simulink model "Adp_Lgt_SytmV2"  (R2021a)
settings: Solver=FixedStepDiscrete  StartTime=0.0  StopTime=1149  FixedStep=1  RelTol=1e-3
libraries: simulink x7
(part 1 of 2)
settings Model: Creator=Akshy  LastModifiedBy=abc
settings OptimizationCC: DefaultParameterBehavior=Inlined  UseDivisionForNetSlopeComputation=on  EnhancedBackFolding=on  PassReuseOutputArgsAs=Individual arguments  ZeroExternalMemoryAtStartup=off  ZeroInternalMemoryAtStartup=off  InitFltsAndDblsToZero=on  OptimizeBlockOrder=speed  DifferentSizesBufferReuse=on  OptimizationCustomize=off  EfficientTunableParamExpr=on
settings DebuggingCC: SignalInfNanChecking=warning  CheckMatrixSingularityMsg=error  IntegerOverflowMsg=error  ParameterTunabilityLossMsg=error  UniqueDataStoreMsg=warning  AssertControl=DisableAll  StrictBusMsg=ErrorOnBusTreatedAsVector  SFUndirectedBroadcastEventsDiag=error  IntegerSaturationMsg=error
settings SFSimCC: CompileTimeRecursionLimit=0  EnableRuntimeRecursion=off  MATLABDynamicMemAlloc=off
settings RTWCC: SystemTargetFile=ert.tlc  GenCodeOnly=on  TemplateMakefile=ert_default_tmf  GenerateReport=on  Toolchain=MinGW64 | gmake (64-bit Windows)  IncludeHyperlinkInReport=on  GenerateTraceInfo=on  GenerateTraceReportSl=on  GenerateTraceReportSf=on
settings CodeAppCC: ForceParamTrailComments=on  IgnoreCustomStorageClasses=off  OperatorAnnotations=on  SimulinkDataObjDesc=on  SFDataObjDesc=on  MATLABFcnDesc=on  InsertBlockDesc=on
settings ERTTargetCC: TargetLangStandard=C99 (ISO)  UtilityFuncGeneration=Shared location  GenerateSampleERTMain=on  SupportAbsoluteTime=off  ParenthesesLevel=Maximum  CastingMode=Standards  GenerateSharedConstants=off  InlinedParameterPlacement=NonHierarchical  ERTCustomFileTemplate=example_file_process.tlc  EnableSignedLeftShifts=off  EnableSignedRightShifts=off
settings ConfigComp: CovMetricSettings=dcmwe  PSVerificationSettings=PrjConfigAndMisraC2012  PSAutoStubLUT=on

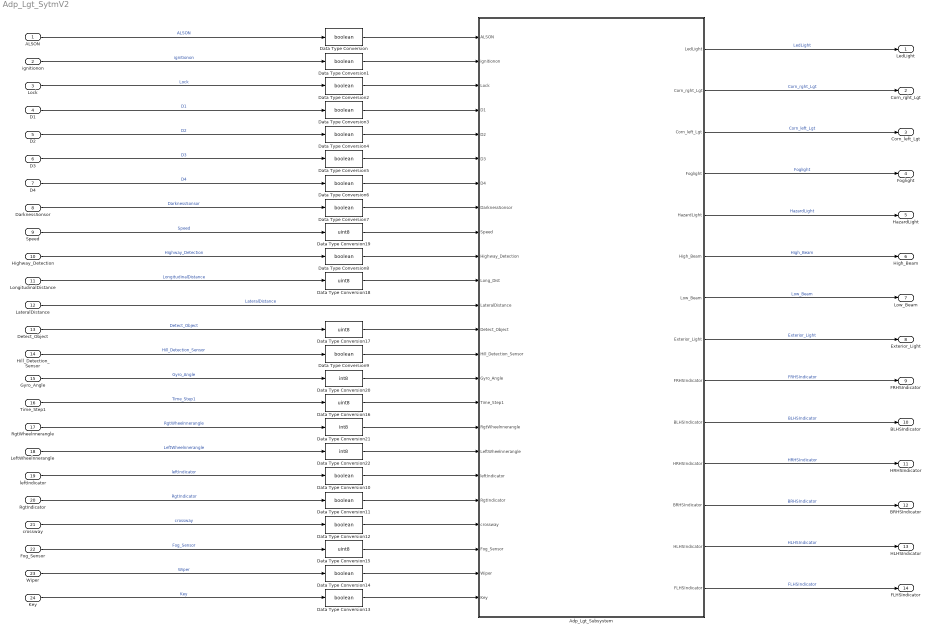
== system Adp_Lgt_SytmV2 ==
  ALSON : Inport
  ignitionon : Inport  Port=2
  Lock : Inport  Port=3
  D1 : Inport  Port=4
  D2 : Inport  Port=5
  D3 : Inport  Port=6
  D4 : Inport  Port=7
  DarknessSonsor : Inport  Port=8
  Speed : Inport  Port=9
  Highway_Detection : Inport  Port=10
  LongitudinalDistance : Inport  Port=11
  LateralDistance : Inport  Port=12
  Detect_Object : Inport  Port=13
  Hill_Detection_Sensor : Inport  Port=14
  Gyro_Angle : Inport  Port=15
  Time_Step1 : Inport  Port=16
  RgtWheelnnerangle : Inport  Port=17
  LeftWheelnnerangle : Inport  Port=18
  leftIndicator : Inport  Port=19
  RgtIndicator : Inport  Port=20
  crossway : Inport  Port=21
  Fog_Sensor : Inport  Port=22
  Wiper : Inport  Port=23
  Key : Inport  Port=24
  Adp_Lgt_Subsystem : Subsystem  TreatAsAtomicUnit=on
  Data Type Conversion{,1..14} (15 alike) : DataTypeConversion  OutDataTypeStr=boolean
  Data Type Conversion{15..19} (5 alike) : DataTypeConversion  OutDataTypeStr=uint8
  Data Type Conversion20 : DataTypeConversion  OutDataTypeStr=int8
  Data Type Conversion21 : DataTypeConversion  OutDataTypeStr=int8
  Data Type Conversion22 : DataTypeConversion  OutDataTypeStr=int8
  LedLight : Outport
  Corn_rght_Lgt : Outport  Port=2
  Corn_left_Lgt : Outport  Port=3
  Foglight : Outport  Port=4
  HazardLight : Outport  Port=5
  High_Beam : Outport  Port=6
  Low_Beam : Outport  Port=7
  Exterior_Light : Outport  Port=8
  FRHSIndicator : Outport  Port=9
  BLHSIndicator : Outport  Port=10
  HRHSIndicator : Outport  Port=11
  BRHSIndicator : Outport  Port=12
  HLHSIndicator : Outport  Port=13
  FLHSIndicator : Outport  Port=14
  wires:
  Adp_Lgt_Subsystem/13(HLHSIndicator) -> HLHSIndicator/1  "HLHSIndicator"
  Adp_Lgt_Subsystem/11(HRHSIndicator) -> HRHSIndicator/1  "HRHSIndicator"
  Adp_Lgt_Subsystem/9(FRHSIndicator) -> FRHSIndicator/1  "FRHSIndicator"
  Adp_Lgt_Subsystem/12(BRHSIndicator) -> BRHSIndicator/1  "BRHSIndicator"
  Adp_Lgt_Subsystem/4(Foglight) -> Foglight/1  "Foglight"
  Adp_Lgt_Subsystem/8(Exterior_Light) -> Exterior_Light/1  "Exterior_Light"
  Adp_Lgt_Subsystem/3(Corn_left_Lgt) -> Corn_left_Lgt/1  "Corn_left_Lgt"
  Adp_Lgt_Subsystem/6(High_Beam) -> High_Beam/1  "High_Beam"
  Adp_Lgt_Subsystem/10(BLHSIndicator) -> BLHSIndicator/1  "BLHSIndicator"
  Adp_Lgt_Subsystem/7(Low_Beam) -> Low_Beam/1  "Low_Beam"
  Adp_Lgt_Subsystem/14(FLHSIndicator) -> FLHSIndicator/1  "FLHSIndicator"
  Adp_Lgt_Subsystem/2(Corn_rght_Lgt) -> Corn_rght_Lgt/1  "Corn_rght_Lgt"
  Adp_Lgt_Subsystem/1(LedLight) -> LedLight/1  "LedLight"
  Adp_Lgt_Subsystem/5(HazardLight) -> HazardLight/1  "HazardLight"
  Data Type Conversion/1 -> Adp_Lgt_Subsystem/1(ALSON)
  Data Type Conversion1/1 -> Adp_Lgt_Subsystem/2(ignitionon)
  Data Type Conversion2/1 -> Adp_Lgt_Subsystem/3(Lock)
  Data Type Conversion3/1 -> Adp_Lgt_Subsystem/4(D1)
  Data Type Conversion4/1 -> Adp_Lgt_Subsystem/5(D2)
  Data Type Conversion5/1 -> Adp_Lgt_Subsystem/6(D3)
  Data Type Conversion6/1 -> Adp_Lgt_Subsystem/7(D4)
  Data Type Conversion7/1 -> Adp_Lgt_Subsystem/8(DarknessSonsor)
  Data Type Conversion8/1 -> Adp_Lgt_Subsystem/10(Highway_Detection)
  Data Type Conversion9/1 -> Adp_Lgt_Subsystem/14(Hill_Detection_Sensor)
  Data Type Conversion10/1 -> Adp_Lgt_Subsystem/19(leftIndicator)
  Data Type Conversion11/1 -> Adp_Lgt_Subsystem/20(RgtIndicator)
  Data Type Conversion12/1 -> Adp_Lgt_Subsystem/21(crossway)
  Data Type Conversion13/1 -> Adp_Lgt_Subsystem/24(Key)
  Data Type Conversion14/1 -> Adp_Lgt_Subsystem/23(Wiper)
  Data Type Conversion15/1 -> Adp_Lgt_Subsystem/22(Fog_Sensor)
  Data Type Conversion16/1 -> Adp_Lgt_Subsystem/16(Time_Step1)
  Data Type Conversion17/1 -> Adp_Lgt_Subsystem/13(Detect_Object)
  Data Type Conversion18/1 -> Adp_Lgt_Subsystem/11(Long_Dist)
  Data Type Conversion19/1 -> Adp_Lgt_Subsystem/9(Speed)
  Data Type Conversion20/1 -> Adp_Lgt_Subsystem/15(Gyro_Angle)
  Data Type Conversion21/1 -> Adp_Lgt_Subsystem/17(RgtWheelnnerangle)
  Data Type Conversion22/1 -> Adp_Lgt_Subsystem/18(LeftWheelnnerangle)
  Detect_Object/1 -> Data Type Conversion17/1  "Detect_Object"
  Time_Step1/1 -> Data Type Conversion16/1  "Time_Step1"
  leftIndicator/1 -> Data Type Conversion10/1  "leftIndicator"
  Wiper/1 -> Data Type Conversion14/1  "Wiper"
  Hill_Detection_Sensor/1 -> Data Type Conversion9/1  "Hill_Detection_Sensor"
  Fog_Sensor/1 -> Data Type Conversion15/1  "Fog_Sensor"
  Gyro_Angle/1 -> Data Type Conversion20/1  "Gyro_Angle"
  crossway/1 -> Data Type Conversion12/1  "crossway"
  LeftWheelnnerangle/1 -> Data Type Conversion22/1  "LeftWheelnnerangle"
  RgtWheelnnerangle/1 -> Data Type Conversion21/1  "RgtWheelnnerangle"
  Highway_Detection/1 -> Data Type Conversion8/1  "Highway_Detection"
  D3/1 -> Data Type Conversion5/1  "D3"
  RgtIndicator/1 -> Data Type Conversion11/1  "RgtIndicator"
  LateralDistance/1 -> Adp_Lgt_Subsystem/12(LateralDistance)  "LateralDistance"
  LongitudinalDistance/1 -> Data Type Conversion18/1  "LongitudinalDistance"
  Lock/1 -> Data Type Conversion2/1  "Lock"
  DarknessSonsor/1 -> Data Type Conversion7/1  "DarknessSonsor"
  ALSON/1 -> Data Type Conversion/1  "ALSON"
  D2/1 -> Data Type Conversion4/1  "D2"
  ignitionon/1 -> Data Type Conversion1/1  "ignitionon"
  D4/1 -> Data Type Conversion6/1  "D4"
  Key/1 -> Data Type Conversion13/1  "Key"
  D1/1 -> Data Type Conversion3/1  "D1"
  Speed/1 -> Data Type Conversion19/1  "Speed"

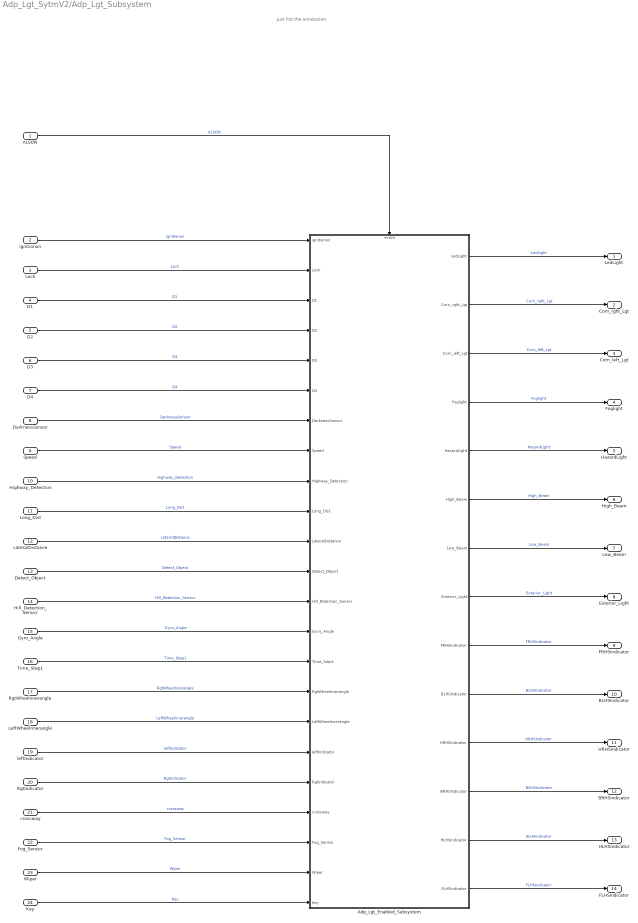
== system Adp_Lgt_SytmV2/Adp_Lgt_Subsystem ==
  note: Just Put the annotation
  ALSON : Inport  OutDataTypeStr=boolean
  ignitionon : Inport  Port=2  OutDataTypeStr=boolean
  Lock : Inport  Port=3  OutDataTypeStr=boolean
  D1 : Inport  Port=4  OutDataTypeStr=boolean
  D2 : Inport  Port=5  OutDataTypeStr=boolean
  D3 : Inport  Port=6  OutDataTypeStr=boolean
  D4 : Inport  Port=7  OutDataTypeStr=boolean
  DarknessSonsor : Inport  Port=8  OutDataTypeStr=boolean
  Speed : Inport  Port=9  OutDataTypeStr=uint8
  Highway_Detection : Inport  Port=10  OutDataTypeStr=boolean
  Long_Dist : Inport  Port=11  OutDataTypeStr=uint8
  LateralDistance : Inport  Port=12  OutDataTypeStr=double
  Detect_Object : Inport  Port=13  OutDataTypeStr=uint8
  Hill_Detection_Sensor : Inport  Port=14  OutDataTypeStr=boolean
  Gyro_Angle : Inport  Port=15  OutDataTypeStr=int8
  Time_Step1 : Inport  Port=16  OutDataTypeStr=uint8
  RgtWheelnnerangle : Inport  Port=17  OutDataTypeStr=int8
  LeftWheelnnerangle : Inport  Port=18  OutDataTypeStr=int8
  leftIndicator : Inport  Port=19  OutDataTypeStr=boolean
  RgtIndicator : Inport  Port=20  OutDataTypeStr=boolean
  crossway : Inport  Port=21  OutDataTypeStr=boolean
  Fog_Sensor : Inport  Port=22  OutDataTypeStr=uint8
  Wiper : Inport  Port=23
  Key : Inport  Port=24  OutDataTypeStr=boolean
  Adp_Lgt_Enabled_Subsystem : Subsystem  TreatAsAtomicUnit=on
  LedLight : Outport
  Corn_rght_Lgt : Outport  Port=2
  Corn_left_Lgt : Outport  Port=3
  Foglight : Outport  Port=4
  HazardLight : Outport  Port=5
  High_Beam : Outport  Port=6
  Low_Beam : Outport  Port=7
  Exterior_Light : Outport  Port=8
  FRHSIndicator : Outport  Port=9
  BLHSIndicator : Outport  Port=10
  HRHSIndicator : Outport  Port=11
  BRHSIndicator : Outport  Port=12
  HLHSIndicator : Outport  Port=13
  FLHSIndicator : Outport  Port=14
  wires:
  LeftWheelnnerangle/1 -> Adp_Lgt_Enabled_Subsystem/17(LeftWheelnnerangle)  "LeftWheelnnerangle"
  Detect_Object/1 -> Adp_Lgt_Enabled_Subsystem/12(Detect_Object)  "Detect_Object"
  D4/1 -> Adp_Lgt_Enabled_Subsystem/6(D4)  "D4"
  RgtWheelnnerangle/1 -> Adp_Lgt_Enabled_Subsystem/16(RgtWheelnnerangle)  "RgtWheelnnerangle"
  LateralDistance/1 -> Adp_Lgt_Enabled_Subsystem/11(LateralDistance)  "LateralDistance"
  Adp_Lgt_Enabled_Subsystem/1(LedLight) -> LedLight/1  "LedLight"
  Adp_Lgt_Enabled_Subsystem/2(Corn_rght_Lgt) -> Corn_rght_Lgt/1  "Corn_rght_Lgt"
  Adp_Lgt_Enabled_Subsystem/4(Foglight) -> Foglight/1  "Foglight"
  crossway/1 -> Adp_Lgt_Enabled_Subsystem/20(crossway)  "crossway"
  RgtIndicator/1 -> Adp_Lgt_Enabled_Subsystem/19(RgtIndicator)  "RgtIndicator"
  Highway_Detection/1 -> Adp_Lgt_Enabled_Subsystem/9(Highway_Detection)  "Highway_Detection"
  leftIndicator/1 -> Adp_Lgt_Enabled_Subsystem/18(leftIndicator)  "leftIndicator"
  DarknessSonsor/1 -> Adp_Lgt_Enabled_Subsystem/7(DarknessSonsor)  "DarknessSonsor"
  ignitionon/1 -> Adp_Lgt_Enabled_Subsystem/1(ignitionon)  "ignitionon"
  Speed/1 -> Adp_Lgt_Enabled_Subsystem/8(Speed)  "Speed"
  Adp_Lgt_Enabled_Subsystem/5(HazardLight) -> HazardLight/1  "HazardLight"
  Time_Step1/1 -> Adp_Lgt_Enabled_Subsystem/15(Time_Step1)  "Time_Step1"
  Fog_Sensor/1 -> Adp_Lgt_Enabled_Subsystem/21(Fog_Sensor)  "Fog_Sensor"
  Lock/1 -> Adp_Lgt_Enabled_Subsystem/2(Lock)  "Lock"
  Long_Dist/1 -> Adp_Lgt_Enabled_Subsystem/10(Long_Dist)  "Long_Dist"
  D1/1 -> Adp_Lgt_Enabled_Subsystem/3(D1)  "D1"
  Gyro_Angle/1 -> Adp_Lgt_Enabled_Subsystem/14(Gyro_Angle)  "Gyro_Angle"
  D3/1 -> Adp_Lgt_Enabled_Subsystem/5(D3)  "D3"
  Wiper/1 -> Adp_Lgt_Enabled_Subsystem/22(Wiper)  "Wiper"
  Adp_Lgt_Enabled_Subsystem/3(Corn_left_Lgt) -> Corn_left_Lgt/1  "Corn_left_Lgt"
  D2/1 -> Adp_Lgt_Enabled_Subsystem/4(D2)  "D2"
  ALSON/1 -> Adp_Lgt_Enabled_Subsystem/Enable  "ALSON"
  Key/1 -> Adp_Lgt_Enabled_Subsystem/23(Key)  "Key"
  Adp_Lgt_Enabled_Subsystem/9(FRHSIndicator) -> FRHSIndicator/1  "FRHSIndicator"
  Adp_Lgt_Enabled_Subsystem/10(BLHSIndicator) -> BLHSIndicator/1  "BLHSIndicator"
  Adp_Lgt_Enabled_Subsystem/11(HRHSIndicator) -> HRHSIndicator/1  "HRHSIndicator"
  Adp_Lgt_Enabled_Subsystem/14(FLHSIndicator) -> FLHSIndicator/1  "FLHSIndicator"
  Adp_Lgt_Enabled_Subsystem/8(Exterior_Light) -> Exterior_Light/1  "Exterior_Light"
  Adp_Lgt_Enabled_Subsystem/12(BRHSIndicator) -> BRHSIndicator/1  "BRHSIndicator"
  Adp_Lgt_Enabled_Subsystem/13(HLHSIndicator) -> HLHSIndicator/1  "HLHSIndicator"
  Adp_Lgt_Enabled_Subsystem/6(High_Beam) -> High_Beam/1  "High_Beam"
  Adp_Lgt_Enabled_Subsystem/7(Low_Beam) -> Low_Beam/1  "Low_Beam"
  Hill_Detection_Sensor/1 -> Adp_Lgt_Enabled_Subsystem/13(Hill_Detection_Sensor)  "Hill_Detection_Sensor"

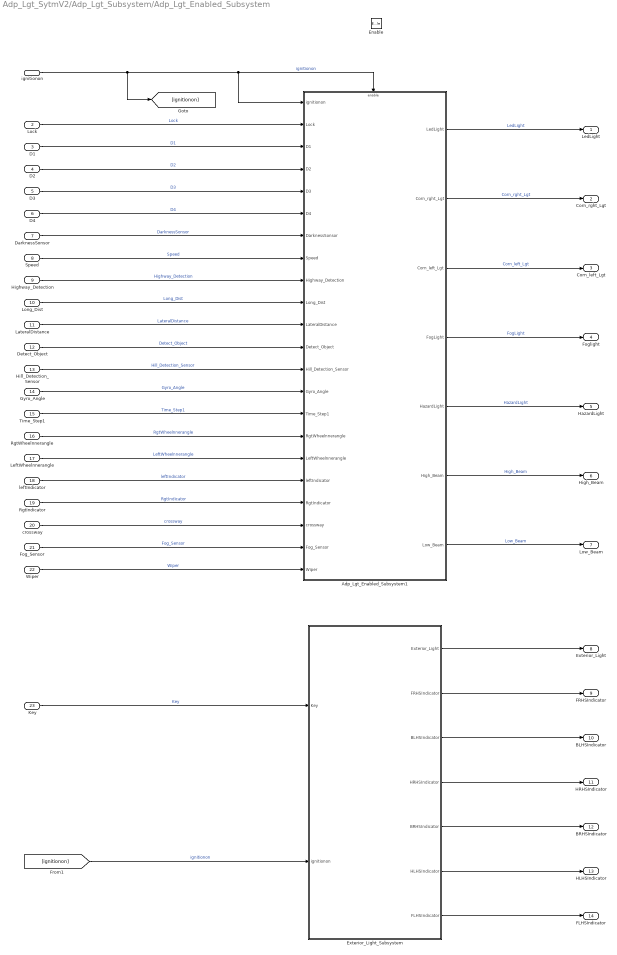
== system Adp_Lgt_SytmV2/Adp_Lgt_Subsystem/Adp_Lgt_Enabled_Subsystem ==
  ignitionon : Inport
  Lock : Inport  Port=2
  D1 : Inport  Port=3
  D2 : Inport  Port=4
  D3 : Inport  Port=5  OutDataTypeStr=boolean
  D4 : Inport  Port=6
  DarknessSonsor : Inport  Port=7
  Speed : Inport  Port=8
  Highway_Detection : Inport  Port=9
  Long_Dist : Inport  Port=10
  LateralDistance : Inport  Port=11
  Detect_Object : Inport  Port=12
  Hill_Detection_Sensor : Inport  Port=13
  Gyro_Angle : Inport  Port=14
  Time_Step1 : Inport  Port=15
  RgtWheelnnerangle : Inport  Port=16
  LeftWheelnnerangle : Inport  Port=17
  leftIndicator : Inport  Port=18
  RgtIndicator : Inport  Port=19
  crossway : Inport  Port=20
  Fog_Sensor : Inport  Port=21  OutDataTypeStr=uint8
  Wiper : Inport  Port=22
  Key : Inport  Port=23
  Enable : EnablePort
  Adp_Lgt_Enabled_Subsystem1 : Subsystem  TreatAsAtomicUnit=on
  Exterior_Light_Subsystem : Subsystem  TreatAsAtomicUnit=on
  LedLight : Outport
  Corn_rght_Lgt : Outport  Port=2
  Corn_left_Lgt : Outport  Port=3
  Foglight : Outport  Port=4
  HazardLight : Outport  Port=5
  High_Beam : Outport  Port=6
  Low_Beam : Outport  Port=7
  Exterior_Light : Outport  Port=8
  FRHSIndicator : Outport  Port=9
  BLHSIndicator : Outport  Port=10
  HRHSIndicator : Outport  Port=11
  BRHSIndicator : Outport  Port=12
  HLHSIndicator : Outport  Port=13
  FLHSIndicator : Outport  Port=14
  wires:
  D4/1 -> Adp_Lgt_Enabled_Subsystem1/6(D4)  "D4"
  DarknessSonsor/1 -> Adp_Lgt_Enabled_Subsystem1/7(DarknessSonsor)  "DarknessSonsor"
  Fog_Sensor/1 -> Adp_Lgt_Enabled_Subsystem1/21(Fog_Sensor)  "Fog_Sensor"
  Wiper/1 -> Adp_Lgt_Enabled_Subsystem1/22(Wiper)  "Wiper"
  D1/1 -> Adp_Lgt_Enabled_Subsystem1/3(D1)  "D1"
  Lock/1 -> Adp_Lgt_Enabled_Subsystem1/2(Lock)  "Lock"
  D2/1 -> Adp_Lgt_Enabled_Subsystem1/4(D2)  "D2"
  D3/1 -> Adp_Lgt_Enabled_Subsystem1/5(D3)  "D3"
  crossway/1 -> Adp_Lgt_Enabled_Subsystem1/20(crossway)  "crossway"
  Speed/1 -> Adp_Lgt_Enabled_Subsystem1/8(Speed)  "Speed"
  Highway_Detection/1 -> Adp_Lgt_Enabled_Subsystem1/9(Highway_Detection)  "Highway_Detection"
  Long_Dist/1 -> Adp_Lgt_Enabled_Subsystem1/10(Long_Dist)  "Long_Dist"
  LateralDistance/1 -> Adp_Lgt_Enabled_Subsystem1/11(LateralDistance)  "LateralDistance"
  Detect_Object/1 -> Adp_Lgt_Enabled_Subsystem1/12(Detect_Object)  "Detect_Object"
  RgtWheelnnerangle/1 -> Adp_Lgt_Enabled_Subsystem1/16(RgtWheelnnerangle)  "RgtWheelnnerangle"
  LeftWheelnnerangle/1 -> Adp_Lgt_Enabled_Subsystem1/17(LeftWheelnnerangle)  "LeftWheelnnerangle"
  leftIndicator/1 -> Adp_Lgt_Enabled_Subsystem1/18(leftIndicator)  "leftIndicator"
  RgtIndicator/1 -> Adp_Lgt_Enabled_Subsystem1/19(RgtIndicator)  "RgtIndicator"
  Adp_Lgt_Enabled_Subsystem1/4(FogLight) -> Foglight/1  "FogLight"
  Adp_Lgt_Enabled_Subsystem1/5(HazardLight) -> HazardLight/1  "HazardLight"
  Adp_Lgt_Enabled_Subsystem1/1(LedLight) -> LedLight/1  "LedLight"
  Adp_Lgt_Enabled_Subsystem1/2(Corn_rght_Lgt) -> Corn_rght_Lgt/1  "Corn_rght_Lgt"
  Adp_Lgt_Enabled_Subsystem1/3(Corn_left_Lgt) -> Corn_left_Lgt/1  "Corn_left_Lgt"
  Gyro_Angle/1 -> Adp_Lgt_Enabled_Subsystem1/14(Gyro_Angle)  "Gyro_Angle"
  Time_Step1/1 -> Adp_Lgt_Enabled_Subsystem1/15(Time_Step1)  "Time_Step1"
  Key/1 -> Exterior_Light_Subsystem/1(Key)  "Key"
  ignitionon/1 -> Adp_Lgt_Enabled_Subsystem1/Enable, Adp_Lgt_Enabled_Subsystem1/1(ignitionon), [ignitionon]  "ignitionon"
  [ignitionon] -> Exterior_Light_Subsystem/2(ignitionon)  "ignitionon"
  Adp_Lgt_Enabled_Subsystem1/6(High_Beam) -> High_Beam/1  "High_Beam"
  Adp_Lgt_Enabled_Subsystem1/7(Low_Beam) -> Low_Beam/1  "Low_Beam"
  Hill_Detection_Sensor/1 -> Adp_Lgt_Enabled_Subsystem1/13(Hill_Detection_Sensor)  "Hill_Detection_Sensor"
  Exterior_Light_Subsystem/1(Exterior_Light) -> Exterior_Light/1
  Exterior_Light_Subsystem/2(FRHSIndicator) -> FRHSIndicator/1
  Exterior_Light_Subsystem/3(BLHSIndicator) -> BLHSIndicator/1
  Exterior_Light_Subsystem/4(HRHSIndicator) -> HRHSIndicator/1
  Exterior_Light_Subsystem/5(BRHSIndicator) -> BRHSIndicator/1
  Exterior_Light_Subsystem/6(HLHSIndicator) -> HLHSIndicator/1
  Exterior_Light_Subsystem/7(FLHSIndicator) -> FLHSIndicator/1

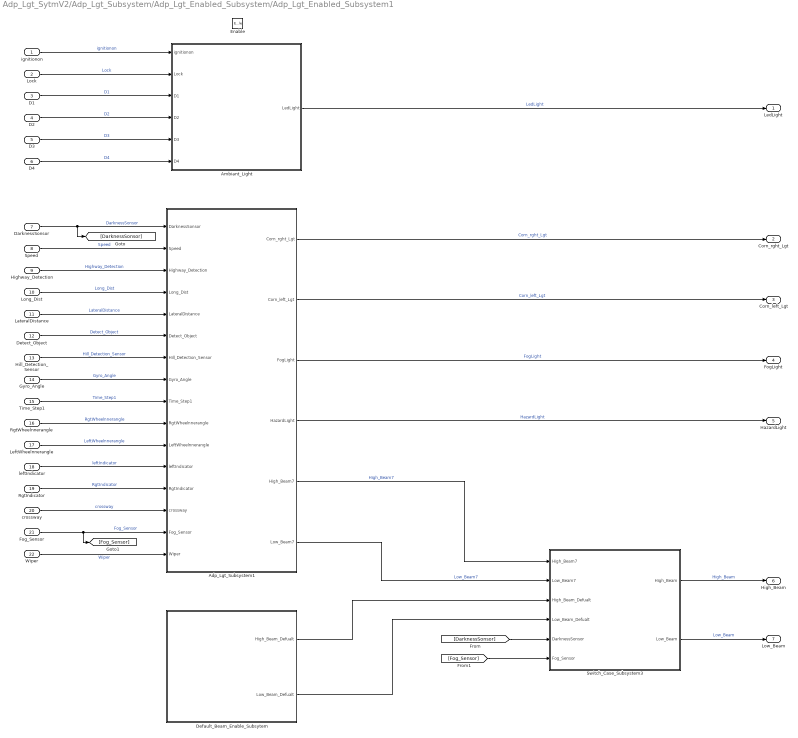
== system Adp_Lgt_SytmV2/Adp_Lgt_Subsystem/Adp_Lgt_Enabled_Subsystem/Adp_Lgt_Enabled_Subsystem1 ==
  ignitionon : Inport
  Lock : Inport  Port=2
  D1 : Inport  Port=3
  D2 : Inport  Port=4
  D3 : Inport  Port=5
  D4 : Inport  Port=6
  DarknessSonsor : Inport  Port=7
  Speed : Inport  Port=8
  Highway_Detection : Inport  Port=9
  Long_Dist : Inport  Port=10
  LateralDistance : Inport  Port=11
  Detect_Object : Inport  Port=12
  Hill_Detection_Sensor : Inport  Port=13
  Gyro_Angle : Inport  Port=14
  Time_Step1 : Inport  Port=15
  RgtWheelnnerangle : Inport  Port=16
  LeftWheelnnerangle : Inport  Port=17
  leftIndicator : Inport  Port=18
  RgtIndicator : Inport  Port=19
  crossway : Inport  Port=20
  Fog_Sensor : Inport  Port=21
  Wiper : Inport  Port=22
  Enable : EnablePort
  Adp_Lgt_Subsystem1 : Subsystem  TreatAsAtomicUnit=on
  Ambiant_Light : Subsystem  TreatAsAtomicUnit=on
  Default_Beam_Enable_Subsytem : Subsystem  TreatAsAtomicUnit=on
  Switch_Case_Subsystem3 : Subsystem  TreatAsAtomicUnit=on
  LedLight : Outport
  Corn_rght_Lgt : Outport  Port=2
  Corn_left_Lgt : Outport  Port=3
  FogLight : Outport  Port=4
  HazardLight : Outport  Port=5
  High_Beam : Outport  Port=6
  Low_Beam : Outport  Port=7
  wires:
  D1/1 -> Ambiant_Light/3(D1)  "D1"
  D3/1 -> Ambiant_Light/5(D3)  "D3"
  D4/1 -> Ambiant_Light/6(D4)  "D4"
  Ambiant_Light/1(LedLight) -> LedLight/1  "LedLight"
  Lock/1 -> Ambiant_Light/2(Lock)  "Lock"
  D2/1 -> Ambiant_Light/4(D2)  "D2"
  ignitionon/1 -> Ambiant_Light/1(ignitionon)  "ignitionon"
  Default_Beam_Enable_Subsytem/2(Low_Beam_Defualt) -> Switch_Case_Subsystem3/4(Low_Beam_Defualt)
  Default_Beam_Enable_Subsytem/1(High_Beam_Defualt) -> Switch_Case_Subsystem3/3(High_Beam_Defualt)
  DarknessSonsor/1 -> [DarknessSonsor], Adp_Lgt_Subsystem1/1(DarknessSonsor)  "DarknessSonsor"
  Speed/1 -> Adp_Lgt_Subsystem1/2(Speed)  "Speed"
  Highway_Detection/1 -> Adp_Lgt_Subsystem1/3(Highway_Detection)  "Highway_Detection"
  Long_Dist/1 -> Adp_Lgt_Subsystem1/4(Long_Dist)  "Long_Dist"
  LateralDistance/1 -> Adp_Lgt_Subsystem1/5(LateralDistance)  "LateralDistance"
  Detect_Object/1 -> Adp_Lgt_Subsystem1/6(Detect_Object)  "Detect_Object"
  Hill_Detection_Sensor/1 -> Adp_Lgt_Subsystem1/7(Hill_Detection_Sensor)  "Hill_Detection_Sensor"
  Gyro_Angle/1 -> Adp_Lgt_Subsystem1/8(Gyro_Angle)  "Gyro_Angle"
  Time_Step1/1 -> Adp_Lgt_Subsystem1/9(Time_Step1)  "Time_Step1"
  RgtWheelnnerangle/1 -> Adp_Lgt_Subsystem1/10(RgtWheelnnerangle)  "RgtWheelnnerangle"
  LeftWheelnnerangle/1 -> Adp_Lgt_Subsystem1/11(LeftWheelnnerangle)  "LeftWheelnnerangle"
  leftIndicator/1 -> Adp_Lgt_Subsystem1/12(leftIndicator)  "leftIndicator"
  RgtIndicator/1 -> Adp_Lgt_Subsystem1/13(RgtIndicator)  "RgtIndicator"
  crossway/1 -> Adp_Lgt_Subsystem1/14(crossway)  "crossway"
  Fog_Sensor/1 -> [Fog_Sensor], Adp_Lgt_Subsystem1/15(Fog_Sensor)  "Fog_Sensor"
  Wiper/1 -> Adp_Lgt_Subsystem1/16(Wiper)  "Wiper"
  Adp_Lgt_Subsystem1/5(High_Beam7) -> Switch_Case_Subsystem3/1(High_Beam7)  "High_Beam7"
  Adp_Lgt_Subsystem1/6(Low_Beam7) -> Switch_Case_Subsystem3/2(Low_Beam7)  "Low_Beam7"
  Adp_Lgt_Subsystem1/1(Corn_rght_Lgt) -> Corn_rght_Lgt/1  "Corn_rght_Lgt"
  Adp_Lgt_Subsystem1/2(Corn_left_Lgt) -> Corn_left_Lgt/1  "Corn_left_Lgt"
  Adp_Lgt_Subsystem1/3(FogLight) -> FogLight/1  "FogLight"
  Adp_Lgt_Subsystem1/4(HazardLight) -> HazardLight/1  "HazardLight"
  [DarknessSonsor] -> Switch_Case_Subsystem3/5(DarknessSonsor)
  [Fog_Sensor] -> Switch_Case_Subsystem3/6(Fog_Sensor)
  Switch_Case_Subsystem3/1(High_Beam) -> High_Beam/1  "High_Beam"
  Switch_Case_Subsystem3/2(Low_Beam) -> Low_Beam/1  "Low_Beam"

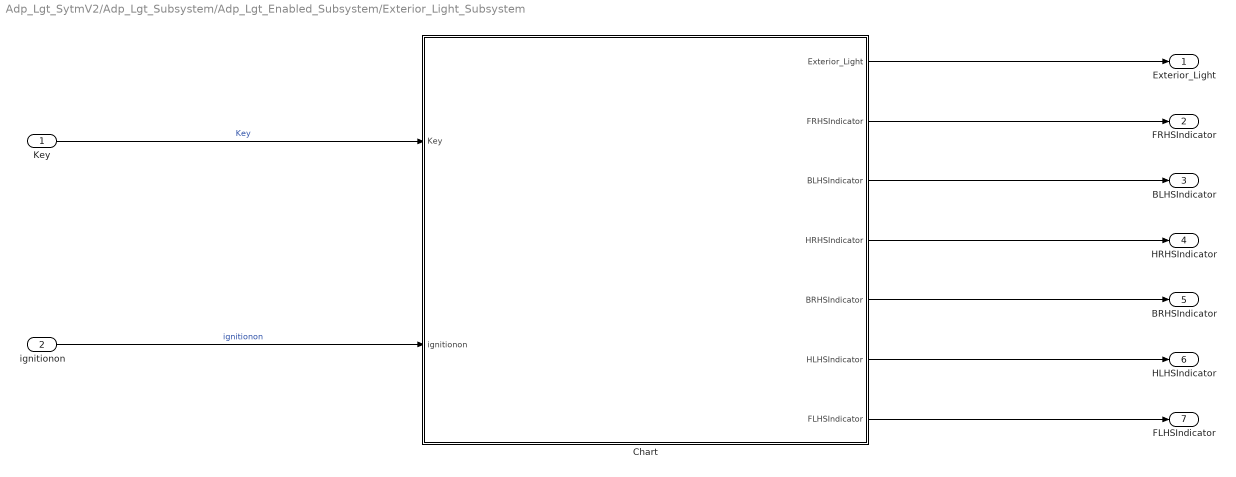
== system Adp_Lgt_SytmV2/Adp_Lgt_Subsystem/Adp_Lgt_Enabled_Subsystem/Exterior_Light_Subsystem ==
  Key : Inport
  ignitionon : Inport  Port=2
  Chart : Stateflow chart  TreatAsAtomicUnit=on
  Exterior_Light : Outport
  FRHSIndicator : Outport  Port=2
  BLHSIndicator : Outport  Port=3
  HRHSIndicator : Outport  Port=4
  BRHSIndicator : Outport  Port=5
  HLHSIndicator : Outport  Port=6
  FLHSIndicator : Outport  Port=7
  wires:
  Chart/6(HLHSIndicator) -> HLHSIndicator/1
  Key/1 -> Chart/1(Key)  "Key"
  Chart/1(Exterior_Light) -> Exterior_Light/1
  Chart/7(FLHSIndicator) -> FLHSIndicator/1
  Chart/2(FRHSIndicator) -> FRHSIndicator/1
  Chart/5(BRHSIndicator) -> BRHSIndicator/1
  Chart/3(BLHSIndicator) -> BLHSIndicator/1
  Chart/4(HRHSIndicator) -> HRHSIndicator/1
  ignitionon/1 -> Chart/2(ignitionon)  "ignitionon"

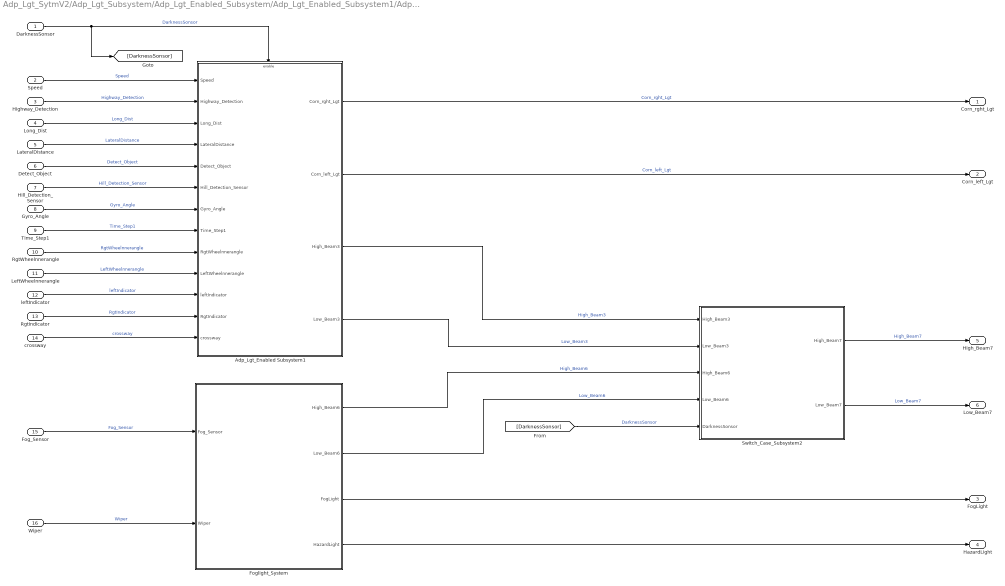
== system Adp_Lgt_SytmV2/Adp_Lgt_Subsystem/Adp_Lgt_Enabled_Subsystem/Adp_Lgt_Enabled_Subsystem1/Adp_Lgt_Subsystem1 ==
  DarknessSonsor : Inport
  Speed : Inport  Port=2
  Highway_Detection : Inport  Port=3
  Long_Dist : Inport  Port=4
  LateralDistance : Inport  Port=5
  Detect_Object : Inport  Port=6
  Hill_Detection_Sensor : Inport  Port=7
  Gyro_Angle : Inport  Port=8
  Time_Step1 : Inport  Port=9
  RgtWheelnnerangle : Inport  Port=10
  LeftWheelnnerangle : Inport  Port=11
  leftIndicator : Inport  Port=12
  RgtIndicator : Inport  Port=13
  crossway : Inport  Port=14
  Fog_Sensor : Inport  Port=15
  Wiper : Inport  Port=16
  Adp_Lgt_Enabled Subsystem1 : Subsystem  TreatAsAtomicUnit=on
  Foglight_System : Subsystem  TreatAsAtomicUnit=on
  Switch_Case_Subsystem2 : Subsystem  TreatAsAtomicUnit=on
  Corn_rght_Lgt : Outport
  Corn_left_Lgt : Outport  Port=2
  FogLight : Outport  Port=3
  HazardLight : Outport  Port=4
  High_Beam7 : Outport  Port=5
  Low_Beam7 : Outport  Port=6
  wires:
  DarknessSonsor/1 -> [DarknessSonsor], Adp_Lgt_Enabled Subsystem1/Enable  "DarknessSonsor"
  RgtIndicator/1 -> Adp_Lgt_Enabled Subsystem1/12(RgtIndicator)  "RgtIndicator"
  Hill_Detection_Sensor/1 -> Adp_Lgt_Enabled Subsystem1/6(Hill_Detection_Sensor)  "Hill_Detection_Sensor"
  Wiper/1 -> Foglight_System/2(Wiper)  "Wiper"
  LateralDistance/1 -> Adp_Lgt_Enabled Subsystem1/4(LateralDistance)  "LateralDistance"
  Highway_Detection/1 -> Adp_Lgt_Enabled Subsystem1/2(Highway_Detection)  "Highway_Detection"
  Fog_Sensor/1 -> Foglight_System/1(Fog_Sensor)  "Fog_Sensor"
  Adp_Lgt_Enabled Subsystem1/3(High_Beam3) -> Switch_Case_Subsystem2/1(High_Beam3)  "High_Beam3"
  Gyro_Angle/1 -> Adp_Lgt_Enabled Subsystem1/7(Gyro_Angle)  "Gyro_Angle"
  Foglight_System/3(FogLight) -> FogLight/1
  Foglight_System/4(HazardLight) -> HazardLight/1
  Detect_Object/1 -> Adp_Lgt_Enabled Subsystem1/5(Detect_Object)  "Detect_Object"
  Long_Dist/1 -> Adp_Lgt_Enabled Subsystem1/3(Long_Dist)  "Long_Dist"
  Time_Step1/1 -> Adp_Lgt_Enabled Subsystem1/8(Time_Step1)  "Time_Step1"
  Speed/1 -> Adp_Lgt_Enabled Subsystem1/1(Speed)  "Speed"
  Adp_Lgt_Enabled Subsystem1/4(Low_Beam3) -> Switch_Case_Subsystem2/2(Low_Beam3)  "Low_Beam3"
  RgtWheelnnerangle/1 -> Adp_Lgt_Enabled Subsystem1/9(RgtWheelnnerangle)  "RgtWheelnnerangle"
  LeftWheelnnerangle/1 -> Adp_Lgt_Enabled Subsystem1/10(LeftWheelnnerangle)  "LeftWheelnnerangle"
  leftIndicator/1 -> Adp_Lgt_Enabled Subsystem1/11(leftIndicator)  "leftIndicator"
  crossway/1 -> Adp_Lgt_Enabled Subsystem1/13(crossway)  "crossway"
  Adp_Lgt_Enabled Subsystem1/2(Corn_left_Lgt) -> Corn_left_Lgt/1  "Corn_left_Lgt"
  Adp_Lgt_Enabled Subsystem1/1(Corn_rght_Lgt) -> Corn_rght_Lgt/1  "Corn_rght_Lgt"
  Foglight_System/2(Low_Beam6) -> Switch_Case_Subsystem2/4(Low_Beam6)  "Low_Beam6"
  Foglight_System/1(High_Beam6) -> Switch_Case_Subsystem2/3(High_Beam6)  "High_Beam6"
  [DarknessSonsor] -> Switch_Case_Subsystem2/5(DarknessSonsor)  "DarknessSonsor"
  Switch_Case_Subsystem2/1(High_Beam7) -> High_Beam7/1  "High_Beam7"
  Switch_Case_Subsystem2/2(Low_Beam7) -> Low_Beam7/1  "Low_Beam7"

== system Adp_Lgt_SytmV2/Adp_Lgt_Subsystem/Adp_Lgt_Enabled_Subsystem/Adp_Lgt_Enabled_Subsystem1/Ambiant_Light ==
  ignitionon : Inport
  Lock : Inport  Port=2
  D1 : Inport  Port=3
  D2 : Inport  Port=4
  D3 : Inport  Port=5  OutDataTypeStr=boolean
  D4 : Inport  Port=6  OutDataTypeStr=boolean
  Chart : Stateflow chart  TreatAsAtomicUnit=on
  OR : Logic  Operator=OR  Inputs=4  AllPortsSameDT=off  OutDataTypeStr=boolean
  LedLight : Outport  OutDataTypeStr=int8
  wires:
  OR/1 -> Chart/3(Lightswitch)  "Lightswitch"
  Lock/1 -> Chart/2(Lock)  "Lock"
  D3/1 -> OR/3  "D3"
  D4/1 -> OR/4  "D4"
  ignitionon/1 -> Chart/1(ignitionon)  "ignitionon"
  Chart/1(LedLight) -> LedLight/1
  D1/1 -> OR/1  "D1"
  D2/1 -> OR/2  "D2"

== system Adp_Lgt_SytmV2/Adp_Lgt_Subsystem/Adp_Lgt_Enabled_Subsystem/Adp_Lgt_Enabled_Subsystem1/Default_Beam_Enable_Subsytem ==
  Chart : Stateflow chart  TreatAsAtomicUnit=on
  High_Beam_Defualt : Outport
  Low_Beam_Defualt : Outport  Port=2
  wires:
  Chart/1(High_Beam_Defualt) -> High_Beam_Defualt/1  "High_Beam_Defualt"
  Chart/2(Low_Beam_Defualt) -> Low_Beam_Defualt/1  "Low_Beam_Defualt"

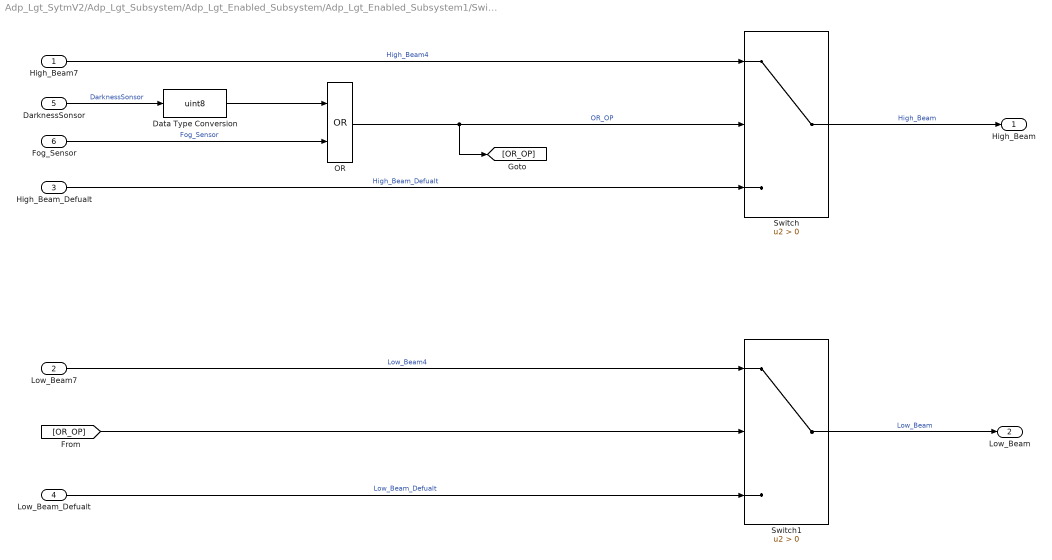
== system Adp_Lgt_SytmV2/Adp_Lgt_Subsystem/Adp_Lgt_Enabled_Subsystem/Adp_Lgt_Enabled_Subsystem1/Switch_Case_Subsystem3 ==
  High_Beam7 : Inport
  Low_Beam7 : Inport  Port=2
  High_Beam_Defualt : Inport  Port=3
  Low_Beam_Defualt : Inport  Port=4
  DarknessSonsor : Inport  Port=5
  Fog_Sensor : Inport  Port=6
  Data Type Conversion : DataTypeConversion  OutDataTypeStr=uint8
  OR : Logic  Operator=OR  AllPortsSameDT=off  OutDataTypeStr=boolean
  Switch : Switch  Criteria=u2 > Threshold
  Switch1 : Switch  Criteria=u2 > Threshold
  High_Beam : Outport
  Low_Beam : Outport  Port=2
  wires:
  Switch/1 -> High_Beam/1  "High_Beam"
  Switch1/1 -> Low_Beam/1  "Low_Beam"
  High_Beam7/1 -> Switch/1  "High_Beam4"
  High_Beam_Defualt/1 -> Switch/3  "High_Beam_Defualt"
  Low_Beam7/1 -> Switch1/1  "Low_Beam4"
  Low_Beam_Defualt/1 -> Switch1/3  "Low_Beam_Defualt"
  DarknessSonsor/1 -> Data Type Conversion/1  "DarknessSonsor"
  Fog_Sensor/1 -> OR/2  "Fog_Sensor"
  OR/1 -> [OR_OP], Switch/2  "OR_OP"
  [OR_OP] -> Switch1/2
  Data Type Conversion/1 -> OR/1

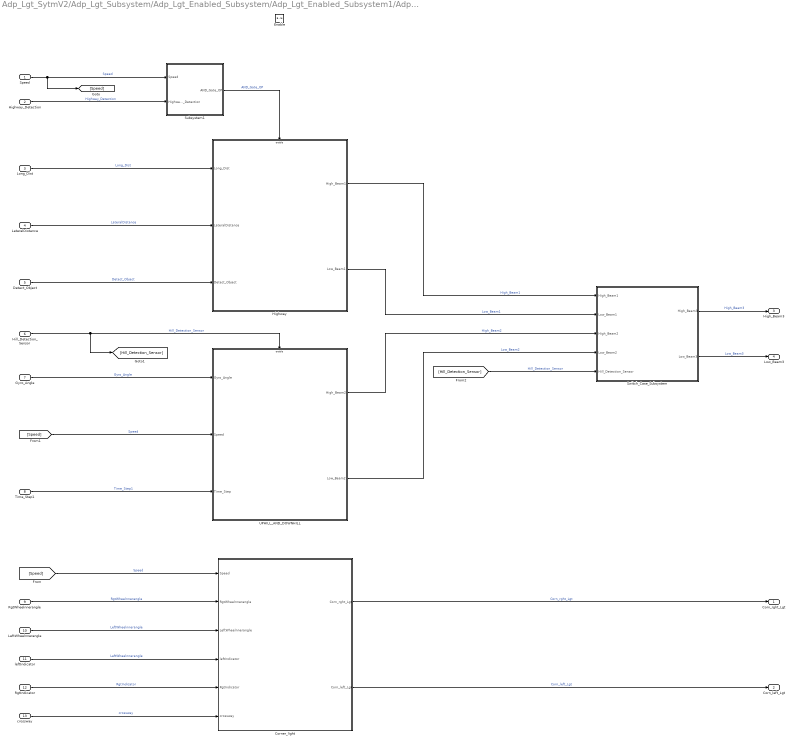
== system Adp_Lgt_SytmV2/Adp_Lgt_Subsystem/Adp_Lgt_Enabled_Subsystem/Adp_Lgt_Enabled_Subsystem1/Adp_Lgt_Subsystem1/Adp_Lgt_Enabled Subsystem1 ==
  Speed : Inport
  Highway_Detection : Inport  Port=2
  Long_Dist : Inport  Port=3
  LateralDistance : Inport  Port=4
  Detect_Object : Inport  Port=5
  Hill_Detection_Sensor : Inport  Port=6
  Gyro_Angle : Inport  Port=7
  Time_Step1 : Inport  Port=8  OutMin=0  OutMax=255  OutDataTypeStr=uint8
  RgtWheelnnerangle : Inport  Port=9
  LeftWheelnnerangle : Inport  Port=10
  leftIndicator : Inport  Port=11
  RgtIndicator : Inport  Port=12
  crossway : Inport  Port=13
  Enable : EnablePort
  Corner_light : Subsystem  TreatAsAtomicUnit=on
  Highway : Subsystem  TreatAsAtomicUnit=on
  Subsystem1 : Subsystem  TreatAsAtomicUnit=on
  Switch_Case_Subsystem : Subsystem  TreatAsAtomicUnit=on
  UPHILL_AND_DOWNHILL : Subsystem  TreatAsAtomicUnit=on
  Corn_rght_Lgt : Outport
  Corn_left_Lgt : Outport  Port=2
  High_Beam3 : Outport  Port=3
  Low_Beam3 : Outport  Port=4
  wires:
  LateralDistance/1 -> Highway/2(LateralDistance)  "LateralDistance"
  Long_Dist/1 -> Highway/1(Long_Dist)  "Long_Dist"
  Highway/2(Low_Beam1) -> Switch_Case_Subsystem/2(Low_Beam1)  "Low_Beam1"
  Highway/1(High_Beam1) -> Switch_Case_Subsystem/1(High_Beam1)  "High_Beam1"
  Detect_Object/1 -> Highway/3(Detect_Object)  "Detect_Object"
  Gyro_Angle/1 -> UPHILL_AND_DOWNHILL/1(Gyro_Angle)  "Gyro_Angle"
  UPHILL_AND_DOWNHILL/2(Low_Beam2) -> Switch_Case_Subsystem/4(Low_Beam2)  "Low_Beam2"
  UPHILL_AND_DOWNHILL/1(High_Beam2) -> Switch_Case_Subsystem/3(High_Beam2)  "High_Beam2"
  Time_Step1/1 -> UPHILL_AND_DOWNHILL/3(Time_Step)  "Time_Step1"
  Speed/1 -> Subsystem1/1(Speed), [Speed]  "Speed"
  [Speed] -> UPHILL_AND_DOWNHILL/2(Speed)  "Speed"
  Corner_light/2(Corn_left_Lgt) -> Corn_left_Lgt/1  "Corn_left_Lgt"
  leftIndicator/1 -> Corner_light/4(leftIndicator)  "LeftWheelnnerangle"
  Corner_light/1(Corn_rght_Lgt) -> Corn_rght_Lgt/1  "Corn_rght_Lgt"
  crossway/1 -> Corner_light/6(crossway)  "crossway"
  RgtIndicator/1 -> Corner_light/5(RgtIndicator)  "RgtIndicator"
  LeftWheelnnerangle/1 -> Corner_light/3(LeftWheelnnerangle)  "LeftWheelnnerangle"
  RgtWheelnnerangle/1 -> Corner_light/2(RgtWheelnnerangle)  "RgtWheelnnerangle"
  [Speed] -> Corner_light/1(Speed)  "Speed"
  Subsystem1/1(AND_Gate_OP) -> Highway/Enable  "AND_Gate_OP"
  Highway_Detection/1 -> Subsystem1/2(Highway_Detection)  "Highway_Detection"
  Hill_Detection_Sensor/1 -> [Hill_Detection_Sensor], UPHILL_AND_DOWNHILL/Enable  "Hill_Detection_Sensor"
  [Hill_Detection_Sensor] -> Switch_Case_Subsystem/5(Hill_Detection_Sensor)  "Hill_Detection_Sensor"
  Switch_Case_Subsystem/1(High_Beam3) -> High_Beam3/1  "High_Beam3"
  Switch_Case_Subsystem/2(Low_Beam3) -> Low_Beam3/1  "Low_Beam3"

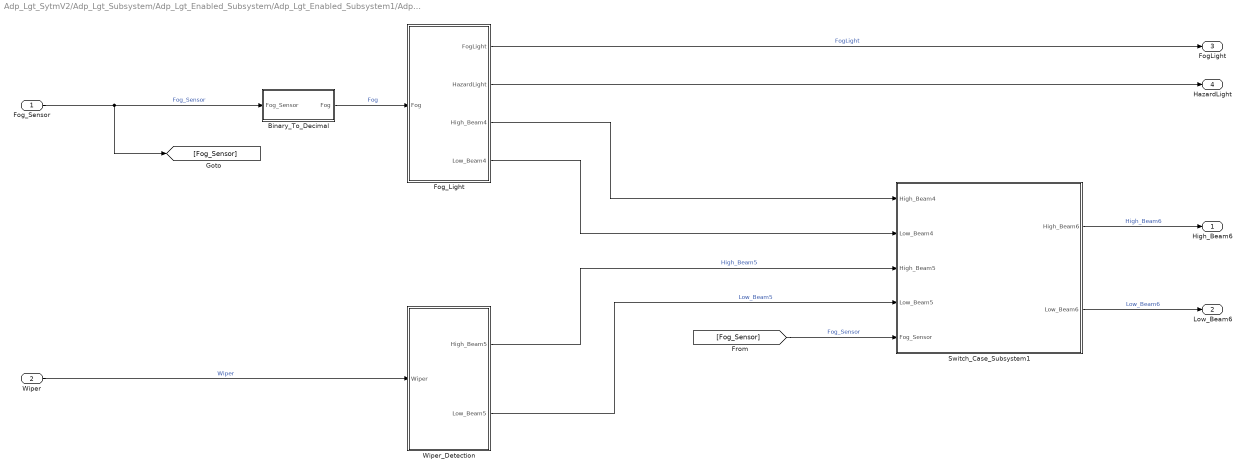
== system Adp_Lgt_SytmV2/Adp_Lgt_Subsystem/Adp_Lgt_Enabled_Subsystem/Adp_Lgt_Enabled_Subsystem1/Adp_Lgt_Subsystem1/Foglight_System ==
  Fog_Sensor : Inport
  Wiper : Inport  Port=2
  Binary_To_Decimal : Subsystem  TreatAsAtomicUnit=on
  Fog_Light : Subsystem  TreatAsAtomicUnit=on
  Switch_Case_Subsystem1 : Subsystem  TreatAsAtomicUnit=on
  Wiper_Detection : Subsystem  TreatAsAtomicUnit=on
  High_Beam6 : Outport
  Low_Beam6 : Outport  Port=2
  FogLight : Outport  Port=3
  HazardLight : Outport  Port=4
  wires:
  Binary_To_Decimal/1(Fog) -> Fog_Light/1(Fog)  "Fog"
  Fog_Light/2(HazardLight) -> HazardLight/1
  Fog_Sensor/1 -> [Fog_Sensor], Binary_To_Decimal/1(Fog_Sensor)  "Fog_Sensor"
  Fog_Light/1(FogLight) -> FogLight/1  "FogLight"
  Fog_Light/3(High_Beam4) -> Switch_Case_Subsystem1/1(High_Beam4)
  Wiper/1 -> Wiper_Detection/1(Wiper)  "Wiper"
  Fog_Light/4(Low_Beam4) -> Switch_Case_Subsystem1/2(Low_Beam4)
  Switch_Case_Subsystem1/1(High_Beam6) -> High_Beam6/1  "High_Beam6"
  Switch_Case_Subsystem1/2(Low_Beam6) -> Low_Beam6/1  "Low_Beam6"
  Wiper_Detection/1(High_Beam5) -> Switch_Case_Subsystem1/3(High_Beam5)  "High_Beam5"
  Wiper_Detection/2(Low_Beam5) -> Switch_Case_Subsystem1/4(Low_Beam5)  "Low_Beam5"
  [Fog_Sensor] -> Switch_Case_Subsystem1/5(Fog_Sensor)  "Fog_Sensor"

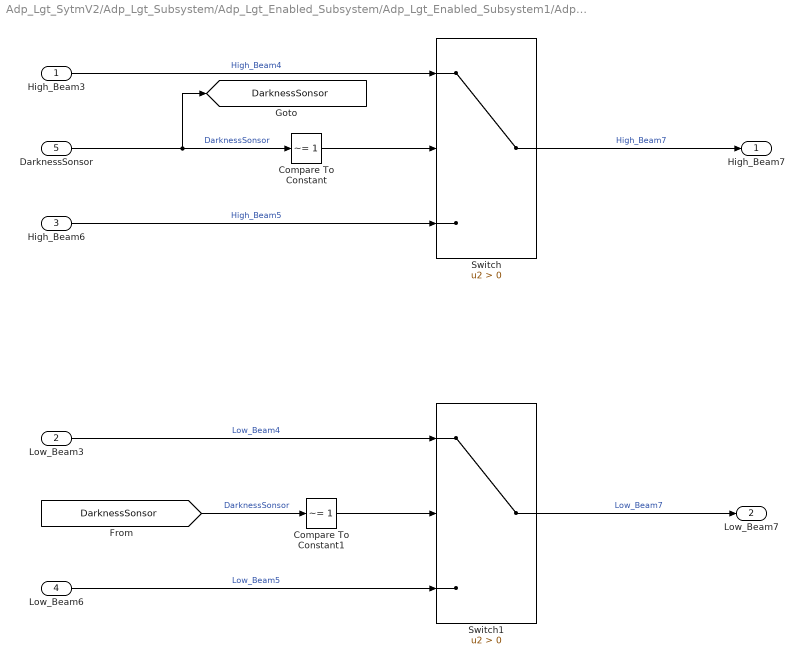
== system Adp_Lgt_SytmV2/Adp_Lgt_Subsystem/Adp_Lgt_Enabled_Subsystem/Adp_Lgt_Enabled_Subsystem1/Adp_Lgt_Subsystem1/Switch_Case_Subsystem2 ==
  High_Beam3 : Inport
  Low_Beam3 : Inport  Port=2
  High_Beam6 : Inport  Port=3
  Low_Beam6 : Inport  Port=4
  DarknessSonsor : Inport  Port=5
  Compare To Constant : simulink/Logic and Bit Operations/Compare To Constant  relop=~=  const=1  OutDataTypeStr=boolean
  Compare To Constant1 : simulink/Logic and Bit Operations/Compare To Constant  relop=~=  const=1  OutDataTypeStr=boolean
  Switch : Switch  Criteria=u2 > Threshold
  Switch1 : Switch  Criteria=u2 > Threshold
  High_Beam7 : Outport
  Low_Beam7 : Outport  Port=2
  tag scope: DarknessSonsor=global
  wires:
  Switch/1 -> High_Beam7/1  "High_Beam7"
  Switch1/1 -> Low_Beam7/1  "Low_Beam7"
  [DarknessSonsor] -> Compare To Constant1/1  "DarknessSonsor"
  DarknessSonsor/1 -> Compare To Constant/1, [DarknessSonsor]  "DarknessSonsor"
  High_Beam3/1 -> Switch/1  "High_Beam4"
  High_Beam6/1 -> Switch/3  "High_Beam5"
  Low_Beam3/1 -> Switch1/1  "Low_Beam4"
  Low_Beam6/1 -> Switch1/3  "Low_Beam5"
  Compare To Constant/1 -> Switch/2
  Compare To Constant1/1 -> Switch1/2

== system Adp_Lgt_SytmV2/Adp_Lgt_Subsystem/Adp_Lgt_Enabled_Subsystem/Adp_Lgt_Enabled_Subsystem1/Adp_Lgt_Subsystem1/Adp_Lgt_Enabled Subsystem1/Corner_light ==
  Speed : Inport
  RgtWheelnnerangle : Inport  Port=2
  LeftWheelnnerangle : Inport  Port=3
  leftIndicator : Inport  Port=4
  RgtIndicator : Inport  Port=5
  crossway : Inport  Port=6
  Chart : Stateflow chart  TreatAsAtomicUnit=on
      settings: PortSchema="{\"entries\":[{\"content\":{\"sides\":[{\"content\":{\"connectorIds\":[\"In3\",\"In2\",\"In1\",\"In4\",\"In5\",\"In6\"]},\"type\":\"ConnectorPlacement.EquallySpacedRectSide\",\"uuid\":\"2620a060-4795-461d-bd09-0b6475982d4d\"},{\"content\":{\"connectorIds\":[\"Out1\",\"Out2\"],\"side\":\"RIGHT\"},\"type\":\"ConnectorPlacement.EquallySpacedRectSide\",\"uuid\":\"407e99ce-bdc2-4ecf-bdaa-040da19bbdfa\"},{\"content\":{\"connectorIds\":[],\"side\":\"TOP\"},\"type\":\"ConnectorPlacement.EquallySpacedRectSide\",\"uuid\":\"c8bfd994-f7e3-4cbc-b36d-612224144721\"}]},\"type\":\"ConnectorPlacement.EquallySpacedConnector\",\"uuid\":\"3980c0f4-0a22-4b32-b618-64ab9315d42b\"}],\"packageUris\":[\"http://schema.mathworks.com/mf0/Connector/R2020b\"],\"version\":\"1.0\"}"
  Corn_rght_Lgt : Outport
  Corn_left_Lgt : Outport  Port=2
  wires:
  RgtIndicator/1 -> Chart/5(RgtIndicator)  "RgtIndicator"
  leftIndicator/1 -> Chart/4(leftIndicator)  "leftIndicator"
  crossway/1 -> Chart/6(crossway)  "crossway"
  Chart/2(Corn_left_Lgt) -> Corn_left_Lgt/1  "Corn_left_Lgt"
  LeftWheelnnerangle/1 -> Chart/1(LeftWheelnnerangle)  "LeftWheelnnerangle"
  RgtWheelnnerangle/1 -> Chart/2(RgtWheelnnerangle)  "RgtWheelnnerangle"
  Chart/1(Corn_rght_Lgt) -> Corn_rght_Lgt/1  "Corn_rght_Lgt"
  Speed/1 -> Chart/3(Speed)  "Speed"

== system Adp_Lgt_SytmV2/Adp_Lgt_Subsystem/Adp_Lgt_Enabled_Subsystem/Adp_Lgt_Enabled_Subsystem1/Adp_Lgt_Subsystem1/Adp_Lgt_Enabled Subsystem1/Highway ==
  Long_Dist : Inport  OutMin=0  OutMax=255  OutDataTypeStr=uint8
  LateralDistance : Inport  Port=2  OutDataTypeStr=double
  Detect_Object : Inport  Port=3
  Enable : EnablePort
  Detect_Object_Enable_Subsystem : Subsystem  TreatAsAtomicUnit=on
  Lane_Detection : Subsystem  TreatAsAtomicUnit=on
  High_Beam1 : Outport
  Low_Beam1 : Outport  Port=2
  wires:
  Long_Dist/1 -> [Long_Dist], Lane_Detection/1(Long_Dist)  "Long_Dist"
  LateralDistance/1 -> Lane_Detection/2(LateralDistance)  "LateralDistance"
  Lane_Detection/1(Left_Lane) -> Detect_Object_Enable_Subsystem/1(Left_Lane)  "Left_Lane"
  [Long_Dist] -> Detect_Object_Enable_Subsystem/3(Long_Dist)  "Long_Dist"
  Detect_Object_Enable_Subsystem/1(High_Beam1) -> High_Beam1/1
  Detect_Object_Enable_Subsystem/2(Low_Beam1) -> Low_Beam1/1
  Detect_Object/1 -> Detect_Object_Enable_Subsystem/2(Detect_Object)  "Detect_Object"

== system Adp_Lgt_SytmV2/Adp_Lgt_Subsystem/Adp_Lgt_Enabled_Subsystem/Adp_Lgt_Enabled_Subsystem1/Adp_Lgt_Subsystem1/Adp_Lgt_Enabled Subsystem1/Subsystem1 ==
  Speed : Inport
  Highway_Detection : Inport  Port=2
  AND : Logic  AllPortsSameDT=off  OutDataTypeStr=boolean
  Compare To Constant : simulink/Logic and Bit Operations/Compare To Constant  relop=>=  const=80  OutDataTypeStr=boolean
  AND_Gate_OP : Outport
  wires:
  AND/1 -> AND_Gate_OP/1  "AND_Gate_OP"
  Speed/1 -> Compare To Constant/1  "Speed"
  Compare To Constant/1 -> AND/1  "Comp_Cons_OP"
  Highway_Detection/1 -> AND/2  "Highway_Detection"

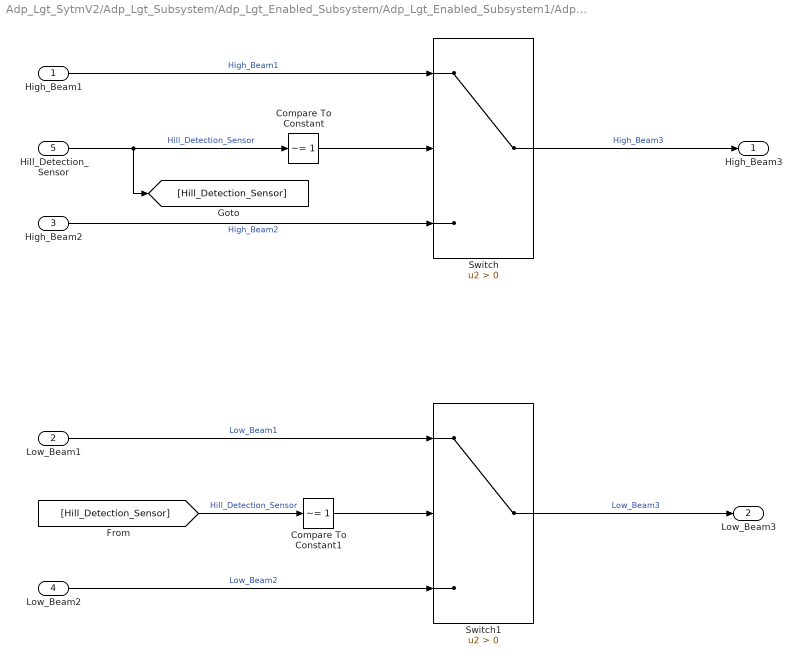
== system Adp_Lgt_SytmV2/Adp_Lgt_Subsystem/Adp_Lgt_Enabled_Subsystem/Adp_Lgt_Enabled_Subsystem1/Adp_Lgt_Subsystem1/Adp_Lgt_Enabled Subsystem1/Switch_Case_Subsystem ==
  High_Beam1 : Inport
  Low_Beam1 : Inport  Port=2
  High_Beam2 : Inport  Port=3
  Low_Beam2 : Inport  Port=4
  Hill_Detection_Sensor : Inport  Port=5
  Compare To Constant : simulink/Logic and Bit Operations/Compare To Constant  relop=~=  const=1  OutDataTypeStr=boolean
  Compare To Constant1 : simulink/Logic and Bit Operations/Compare To Constant  relop=~=  const=1  OutDataTypeStr=boolean
  Switch : Switch  Criteria=u2 > Threshold
  Switch1 : Switch  Criteria=u2 > Threshold
  High_Beam3 : Outport
  Low_Beam3 : Outport  Port=2
  wires:
  Switch/1 -> High_Beam3/1  "High_Beam3"
  Switch1/1 -> Low_Beam3/1  "Low_Beam3"
  [Hill_Detection_Sensor] -> Compare To Constant1/1  "Hill_Detection_Sensor"
  Hill_Detection_Sensor/1 -> [Hill_Detection_Sensor], Compare To Constant/1  "Hill_Detection_Sensor"
  High_Beam1/1 -> Switch/1  "High_Beam1"
  High_Beam2/1 -> Switch/3  "High_Beam2"
  Low_Beam1/1 -> Switch1/1  "Low_Beam1"
  Low_Beam2/1 -> Switch1/3  "Low_Beam2"
  Compare To Constant/1 -> Switch/2
  Compare To Constant1/1 -> Switch1/2

== system Adp_Lgt_SytmV2/Adp_Lgt_Subsystem/Adp_Lgt_Enabled_Subsystem/Adp_Lgt_Enabled_Subsystem1/Adp_Lgt_Subsystem1/Adp_Lgt_Enabled Subsystem1/UPHILL_AND_DOWNHILL ==
  Gyro_Angle : Inport  OutDataTypeStr=int8
  Speed : Inport  Port=2
  Time_Step : Inport  Port=3
  Enable : EnablePort
  Chart : Stateflow chart  TreatAsAtomicUnit=on
  High_Beam2 : Outport
  Low_Beam2 : Outport  Port=2
  wires:
  Time_Step/1 -> Chart/3(Time_Step)
  Speed/1 -> Chart/2(Speed)
  Chart/2(Low_Beam2) -> Low_Beam2/1
  Gyro_Angle/1 -> Chart/1(Gyro_Angle)
  Chart/1(High_Beam2) -> High_Beam2/1

== system Adp_Lgt_SytmV2/Adp_Lgt_Subsystem/Adp_Lgt_Enabled_Subsystem/Adp_Lgt_Enabled_Subsystem1/Adp_Lgt_Subsystem1/Foglight_System/Binary_To_Decimal ==
  Fog_Sensor : Inport  OutDataTypeStr=uint8
  1-D Lookup Table : Lookup_n-D  NumberOfTableDimensions=1  BreakpointsForDimension1=[00 01 10 11]  Table=[0 1 2 3]  ExtrapMethod=Clip  InternalRulePriority=Speed  RndMeth=Simplest  InputSameDT=on
      settings: AttributesFormatString=RndMeth=%<RndMeth>
  Fog : Outport
  wires:
  Fog_Sensor/1 -> 1-D Lookup Table/1  "Fog_Sensor"
  1-D Lookup Table/1 -> Fog/1  "Fog"

== system Adp_Lgt_SytmV2/Adp_Lgt_Subsystem/Adp_Lgt_Enabled_Subsystem/Adp_Lgt_Enabled_Subsystem1/Adp_Lgt_Subsystem1/Foglight_System/Fog_Light ==
  Fog : Inport
  Chart : Stateflow chart  TreatAsAtomicUnit=on
  FogLight : Outport
  HazardLight : Outport  Port=2
  High_Beam4 : Outport  Port=3
  Low_Beam4 : Outport  Port=4
  wires:
  Fog/1 -> Chart/1(Fog)
  Chart/1(FogLight) -> FogLight/1  "FogLight"
  Chart/2(HazardLight) -> HazardLight/1
  Chart/3(High_Beam4) -> High_Beam4/1
  Chart/4(Low_Beam4) -> Low_Beam4/1

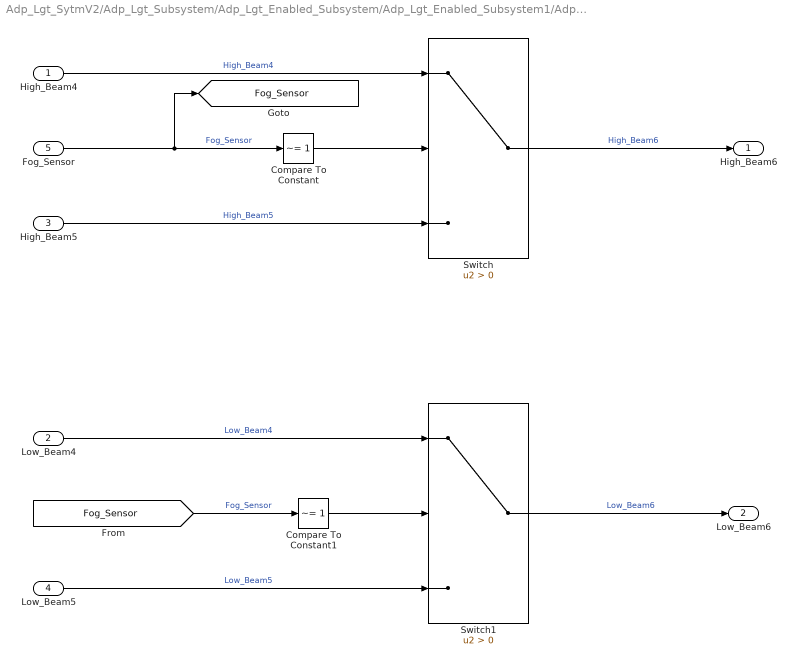
== system Adp_Lgt_SytmV2/Adp_Lgt_Subsystem/Adp_Lgt_Enabled_Subsystem/Adp_Lgt_Enabled_Subsystem1/Adp_Lgt_Subsystem1/Foglight_System/Switch_Case_Subsystem1 ==
  High_Beam4 : Inport
  Low_Beam4 : Inport  Port=2
  High_Beam5 : Inport  Port=3
  Low_Beam5 : Inport  Port=4
  Fog_Sensor : Inport  Port=5
  Compare To Constant : simulink/Logic and Bit Operations/Compare To Constant  relop=~=  const=1  OutDataTypeStr=boolean
  Compare To Constant1 : simulink/Logic and Bit Operations/Compare To Constant  relop=~=  const=1  OutDataTypeStr=boolean
  Switch : Switch  Criteria=u2 > Threshold
  Switch1 : Switch  Criteria=u2 > Threshold
  High_Beam6 : Outport
  Low_Beam6 : Outport  Port=2
  tag scope: Fog_Sensor=global
  wires:
  Switch/1 -> High_Beam6/1  "High_Beam6"
  Switch1/1 -> Low_Beam6/1  "Low_Beam6"
  [Fog_Sensor] -> Compare To Constant1/1  "Fog_Sensor"
  Fog_Sensor/1 -> Compare To Constant/1, [Fog_Sensor]  "Fog_Sensor"
  High_Beam4/1 -> Switch/1  "High_Beam4"
  High_Beam5/1 -> Switch/3  "High_Beam5"
  Low_Beam4/1 -> Switch1/1  "Low_Beam4"
  Low_Beam5/1 -> Switch1/3  "Low_Beam5"
  Compare To Constant/1 -> Switch/2
  Compare To Constant1/1 -> Switch1/2

== system Adp_Lgt_SytmV2/Adp_Lgt_Subsystem/Adp_Lgt_Enabled_Subsystem/Adp_Lgt_Enabled_Subsystem1/Adp_Lgt_Subsystem1/Foglight_System/Wiper_Detection ==
  Wiper : Inport
  Chart : Stateflow chart  TreatAsAtomicUnit=on
  High_Beam5 : Outport
  Low_Beam5 : Outport  Port=2
  wires:
  Chart/2(Low_Beam5) -> Low_Beam5/1  "Low_Beam5"
  Wiper/1 -> Chart/1(Wiper)  "Wiper"
  Chart/1(High_Beam5) -> High_Beam5/1  "High_Beam5"

== system Adp_Lgt_SytmV2/Adp_Lgt_Subsystem/Adp_Lgt_Enabled_Subsystem/Adp_Lgt_Enabled_Subsystem1/Adp_Lgt_Subsystem1/Adp_Lgt_Enabled Subsystem1/Highway/Detect_Object_Enable_Subsystem ==
  Left_Lane : Inport  OutDataTypeStr=uint8
  Detect_Object : Inport  Port=2
  Long_Dist : Inport  Port=3
  Chart : Stateflow chart  TreatAsAtomicUnit=on
      settings: PortSchema="{\"entries\":[{\"content\":{\"sides\":[{\"content\":{\"connectorIds\":[\"In1\",\"In3\",\"In2\"]},\"type\":\"ConnectorPlacement.EquallySpacedRectSide\",\"uuid\":\"91bad8fe-4a08-442f-90ec-8dd30ed61c76\"},{\"content\":{\"connectorIds\":[\"Out1\",\"Out2\"],\"side\":\"RIGHT\"},\"type\":\"ConnectorPlacement.EquallySpacedRectSide\",\"uuid\":\"5d396e88-0832-4a93-a2c1-79594b3f391a\"},{\"content\":{\"connectorIds\":[],\"side\":\"TOP\"},\"type\":\"ConnectorPlacement.EquallySpacedRectSide\",\"uuid\":\"d9453455-17a0-40b0-80d4-03144a3eecad\"}]},\"type\":\"ConnectorPlacement.EquallySpacedConnector\",\"uuid\":\"27d81fd3-d205-4ec6-bb8c-1edcdfcf4177\"}],\"packageUris\":[\"http://schema.mathworks.com/mf0/Connector/R2020b\"],\"version\":\"1.0\"}"
  High_Beam1 : Outport
  Low_Beam1 : Outport  Port=2
  wires:
  Left_Lane/1 -> Chart/1(Left_Lane)
  Chart/2(Low_Beam1) -> Low_Beam1/1  "Low_Beam1"
  Detect_Object/1 -> Chart/3(Detect_Object)
  Chart/1(High_Beam1) -> High_Beam1/1  "High_Beam1"
  Long_Dist/1 -> Chart/2(Long_Dist)

== system Adp_Lgt_SytmV2/Adp_Lgt_Subsystem/Adp_Lgt_Enabled_Subsystem/Adp_Lgt_Enabled_Subsystem1/Adp_Lgt_Subsystem1/Adp_Lgt_Enabled Subsystem1/Highway/Lane_Detection ==
  Long_Dist : Inport
  LateralDistance : Inport  Port=2
  Chart : Stateflow chart  TreatAsAtomicUnit=on
      settings: PortSchema="{\"entries\":[{\"content\":{\"sides\":[{\"content\":{\"connectorIds\":[\"In2\",\"In1\"]},\"type\":\"ConnectorPlacement.EquallySpacedRectSide\",\"uuid\":\"45afa994-8739-48dc-84e8-b1a0f1c0cd9e\"},{\"content\":{\"connectorIds\":[\"Out1\"],\"side\":\"RIGHT\"},\"type\":\"ConnectorPlacement.EquallySpacedRectSide\",\"uuid\":\"9fd1610a-7f7d-46f1-8d6b-b26c50393e15\"},{\"content\":{\"connectorIds\":[],\"side\":\"TOP\"},\"type\":\"ConnectorPlacement.EquallySpacedRectSide\",\"uuid\":\"c0224435-3833-4ecf-8e99-c8ba638dd7b8\"}]},\"type\":\"ConnectorPlacement.EquallySpacedConnector\",\"uuid\":\"ac72c16a-7de8-497e-a625-07d6eb782101\"}],\"packageUris\":[\"http://schema.mathworks.com/mf0/Connector/R2020b\"],\"version\":\"1.0\"}"
  Left_Lane : Outport
  wires:
  LateralDistance/1 -> Chart/1(LateralDistance)  "LateralDistance"
  Long_Dist/1 -> Chart/2(Long_Dist)  "Long_Dist"
  Chart/1(Left_Lane) -> Left_Lane/1  "Left_Lane"

== stateflow chart Adp_Lgt_SytmV2/Adp_Lgt_Subsystem/Adp_Lgt_Enabled_Subsystem/Adp_Lgt_Enabled_Subsystem1/Adp_Lgt_Subsystem1/Adp_Lgt_Enabled Subsystem1/Corner_light/Chart ==
  settings: updateMethod=DISCRETE  sampleTime=1
  state Corner_Light_Default_State
    en:
    Corn_rght_Lgt=0;
    Corn_left_Lgt=0;
  state Corner_Right_Light
    en:
    Corn_rght_Lgt=1;
  state Corner_Left_Light1
    en:
    Corn_left_Lgt=1;
  state Crossing_Line
    en:
    Corn_rght_Lgt=1;
    Corn_left_Lgt=1;
  state Corner_Right_Light1
    en:
    Corn_rght_Lgt=1;
  state Corner_Left_Light2
    en:
    Corn_left_Lgt=1;
  (default) -> Corner_Light_Default_State
  Corner_Light_Default_State -> Corner_Right_Light [order 1] : [((Speed<=20)&&(RgtWheelnnerangle>=5)&&(RgtIndicator==1))]
  Corner_Right_Light -> Corner_Light_Default_State : [(RgtWheelnnerangle<=2)]
  Corner_Light_Default_State -> Corner_Left_Light1 [order 2] : [((Speed<=20)&&(LeftWheelnnerangle<=5)&&(leftIndicator==1))]
  Corner_Left_Light1 -> Corner_Light_Default_State : [(LeftWheelnnerangle<=2)]
  Corner_Light_Default_State -> Crossing_Line [order 3] : [((Speed<=20)&&(crossway==1))]
  Crossing_Line -> Corner_Light_Default_State : [(crossway==0)]
  Corner_Light_Default_State -> Corner_Right_Light1 [order 4] : [((Speed>=80)&&(RgtWheelnnerangle>=5))]
  Corner_Right_Light1 -> Corner_Light_Default_State : [(RgtWheelnnerangle<=2)]
  Corner_Light_Default_State -> Corner_Left_Light2 [order 5] : [((Speed>=80)&&(LeftWheelnnerangle<=5))]
  Corner_Left_Light2 -> Corner_Light_Default_State : [(LeftWheelnnerangle<=2)]
  data: LeftWheelnnerangle input int8; RgtWheelnnerangle input int8; Corn_rght_Lgt output; Corn_left_Lgt output; Speed input uint8; leftIndicator input boolean; RgtIndicator input boolean; crossway input boolean
